simulink library "bus_stubs_fsw"  (R2016b)
settings: Solver=VariableStepAuto  StartTime=0.0  StopTime=10.0  RelTol=1e-3
settings Model: Creator=taylorreynolds  LastModifiedBy=taylorreynolds

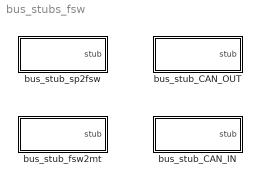
== system bus_stubs_fsw ==
  bus_stub_CAN_IN : Subsystem
      mask help: Creates bus compliant with actuatorCmd (actuator command) bus object.
      mask Help: Provides a zeroed bus which complies with the actuatorCmd bus object.
      mask DialogControl DescGroupVar Prompt: bus_stub_actCmd
      mask DialogControl DescTextVar Prompt: Creates bus compliant with actuatorCmd (actuator command) bus object.
  bus_stub_CAN_OUT : Subsystem
      mask help: Creates bus compliant with actuatorCmd (actuator command) bus object.
      mask Help: Provides a zeroed bus which complies with the actuatorCmd bus object.
      mask DialogControl DescGroupVar Prompt: bus_stub_actCmd
      mask DialogControl DescTextVar Prompt: Creates bus compliant with actuatorCmd (actuator command) bus object.
  bus_stub_fsw2mt : Subsystem
      mask help: Creates bus compliant with actuatorCmd (actuator command) bus object.
      mask Help: Provides a zeroed bus which complies with the actuatorCmd bus object.
      mask DialogControl DescGroupVar Prompt: bus_stub_actCmd
      mask DialogControl DescTextVar Prompt: Creates bus compliant with actuatorCmd (actuator command) bus object.
  bus_stub_sp2fsw : Subsystem
      mask help: Creates bus compliant with actuatorCmd (actuator command) bus object.
      mask Help: Provides a zeroed bus which complies with the actuatorCmd bus object.
      mask DialogControl DescGroupVar Prompt: bus_stub_actCmd
      mask DialogControl DescTextVar Prompt: Creates bus compliant with actuatorCmd (actuator command) bus object.

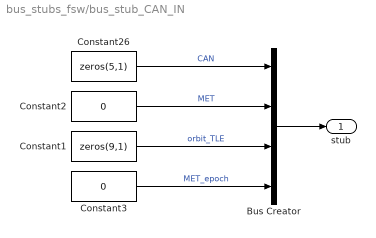
== system bus_stubs_fsw/bus_stub_CAN_IN ==
  Bus Creator : BusCreator  Inputs=4
  Constant1 : Constant  Value=zeros(9,1)
  Constant2 : Constant  Value=0
  Constant26 : Constant  Value=zeros(5,1)  OutDataTypeStr=int8
  Constant3 : Constant  Value=0
  stub : Outport  OutDataTypeStr=Bus: CAN_IN
  wires:
  Constant26/1 -> Bus Creator/1  "CAN"
  Bus Creator/1 -> stub/1
  Constant1/1 -> Bus Creator/3  "orbit_TLE"
  Constant2/1 -> Bus Creator/2  "MET"
  Constant3/1 -> Bus Creator/4  "MET_epoch"

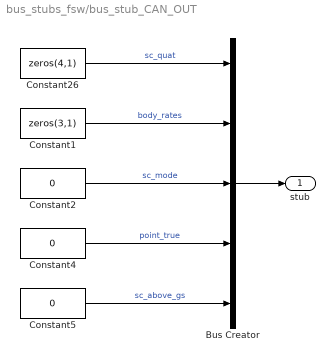
== system bus_stubs_fsw/bus_stub_CAN_OUT ==
  Bus Creator : BusCreator  Inputs=5
  Constant1 : Constant  Value=zeros(3,1)
  Constant2 : Constant  Value=0  OutDataTypeStr=int8
  Constant26 : Constant  Value=zeros(4,1)
  Constant4 : Constant  Value=0  OutDataTypeStr=boolean
  Constant5 : Constant  Value=0  OutDataTypeStr=boolean
  stub : Outport  OutDataTypeStr=Bus: CAN_OUT
  wires:
  Constant26/1 -> Bus Creator/1  "sc_quat"
  Bus Creator/1 -> stub/1
  Constant1/1 -> Bus Creator/2  "body_rates"
  Constant2/1 -> Bus Creator/3  "sc_mode"
  Constant4/1 -> Bus Creator/4  "point_true"
  Constant5/1 -> Bus Creator/5  "sc_above_gs"

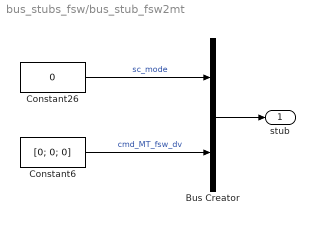
== system bus_stubs_fsw/bus_stub_fsw2mt ==
  Bus Creator : BusCreator  Inputs=2
  Constant26 : Constant  Value=0  OutDataTypeStr=int8
  Constant6 : Constant  Value=[0; 0; 0]  OutDataTypeStr=int8
  stub : Outport  OutDataTypeStr=Bus: fsw2mt
  wires:
  Constant26/1 -> Bus Creator/1  "sc_mode"
  Constant6/1 -> Bus Creator/2  "cmd_MT_fsw_dv"
  Bus Creator/1 -> stub/1

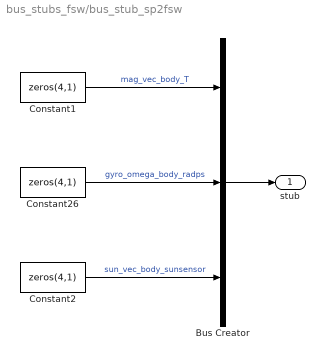
== system bus_stubs_fsw/bus_stub_sp2fsw ==
  Bus Creator : BusCreator  Inputs=3
  Constant1 : Constant  Value=zeros(4,1)  OutDataTypeStr=single
  Constant2 : Constant  Value=zeros(4,1)  OutDataTypeStr=single
  Constant26 : Constant  Value=zeros(4,1)  OutDataTypeStr=single
  stub : Outport  OutDataTypeStr=Bus: sp2fsw
  wires:
  Bus Creator/1 -> stub/1
  Constant26/1 -> Bus Creator/2  "gyro_omega_body_radps"
  Constant1/1 -> Bus Creator/1  "mag_vec_body_T"
  Constant2/1 -> Bus Creator/3  "sun_vec_body_sunsensor"
